simulink model "lump_model_v9"  (R2024b)
settings: Solver=FixedStepAuto  StartTime=0.0  StopTime=100  FixedStep=0.001  RelTol=1e-3
model workspace (MAT data in the model file):
  A_busbar = 0.0015
  A_pack = 0.711626248
  C_nominal = 3
  I_max = 157.708978328
  P = 5
  S = 138
  SoC_initial = 0.78
  T_amb = 297.15
  W_max = 34
  busbar_CC_area = 0.000108
  busbar_Cp = 237
  busbar_length = 0.032
  busbar_mass = 0.01
  busbar_resistivity = 1.68e-08
  busbar_thermalcontact_resistance = 1
  cell_Cp = 1000
  cell_mass = 0.046
  h_busbar = 5
  h_pack = 5
libraries: nesl_utility x8, fl_lib x6, ee_lib x2
settings Model: Creator=kara.28  LastModifiedBy=account

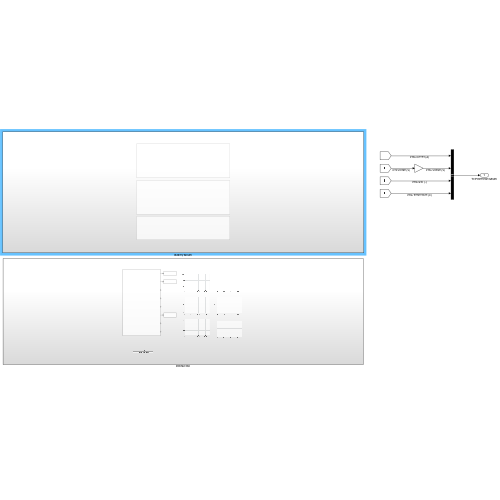
[thumbnail: Simulink's stored preview of the top-level diagram]
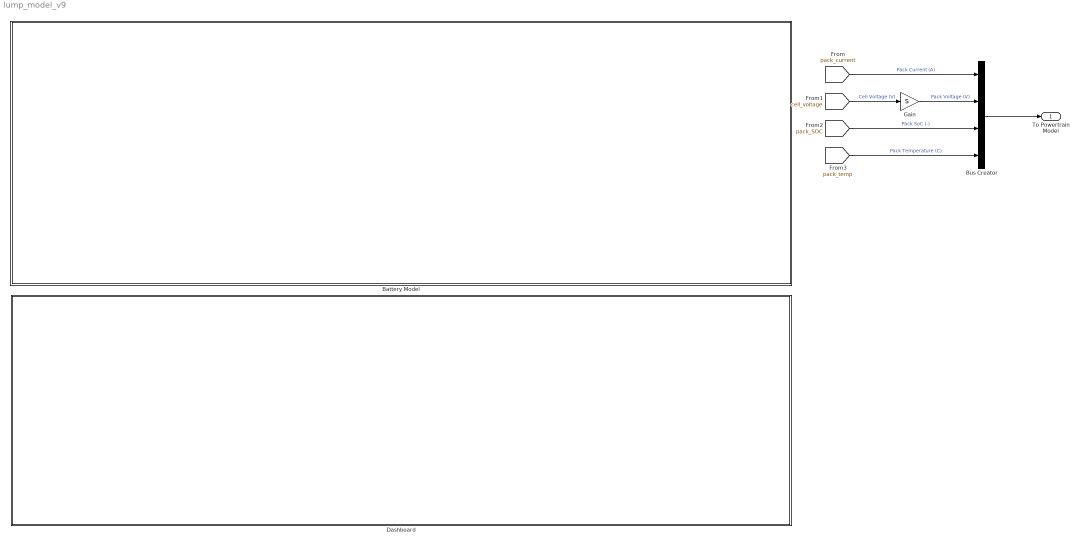
== system lump_model_v9 ==
  Battery Model : Subsystem
  Bus Creator : BusCreator  Inputs=4
  Dashboard : Subsystem
  Gain : Gain  Gain=S
  To Powertrain Model : Outport
  wires:
  [pack_temp] -> Bus Creator/4  "Pack Temperature (C)"
  [pack_SOC] -> Bus Creator/3  "Pack SoC (-)"
  [cell_voltage] -> Gain/1  "Cell Voltage (V)"
  [pack_current] -> Bus Creator/1  "Pack Current (A)"
  Gain/1 -> Bus Creator/2  "Pack Voltage (V)"
  Bus Creator/1 -> To Powertrain Model/1

== system lump_model_v9/Battery Model ==
  Air Temp : Subsystem
  Battery Cells : Subsystem
  Bus Bars : Subsystem

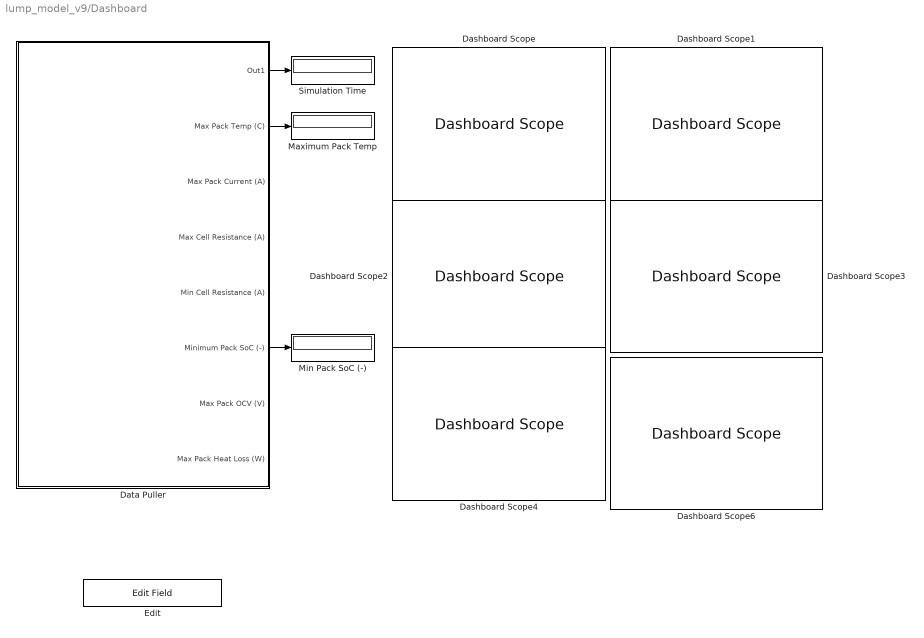
== system lump_model_v9/Dashboard ==
  Dashboard Scope : DashboardScope  Ymin=35  Ymax=60
  Dashboard Scope1 : DashboardScope  Ymin=0  Ymax=180
  Dashboard Scope2 : DashboardScope
  Dashboard Scope3 : DashboardScope  Ymin=0  Ymax=1
  Dashboard Scope4 : DashboardScope  Ymin=2.5  Ymax=4.2
  Dashboard Scope6 : DashboardScope
  Data Puller : Subsystem
  Edit : EditField  ShowInitialText=on  Alignment=Center
  Maximum Pack Temp : Display
  Min Pack SoC (-) : Display
  Simulation Time : Display
  wires:
  Data Puller/1(Out1) -> Simulation Time/1
  Data Puller/2(Max Pack Temp (C)) -> Maximum Pack Temp/1
  Data Puller/6(Minimum Pack SoC (-)) -> Min Pack SoC (-)/1

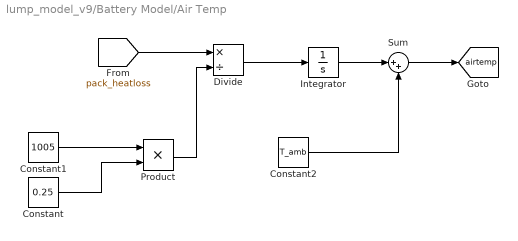
== system lump_model_v9/Battery Model/Air Temp ==
  Constant : Constant  Value=0.25
  Constant1 : Constant  Value=1005
  Constant2 : Constant  Value=T_amb
  Divide : Product  Inputs=*/
  Integrator : Integrator
  Product : Product
  Sum : Sum  Inputs=|++
  tag scope: airtemp=global
  wires:
  [pack_heatloss] -> Divide/1
  Product/1 -> Divide/2
  Constant/1 -> Product/2
  Constant1/1 -> Product/1
  Divide/1 -> Integrator/1
  Integrator/1 -> Sum/1
  Constant2/1 -> Sum/2
  Sum/1 -> [airtemp]

== system lump_model_v9/Battery Model/Battery Cells ==
  Battery Heat : Subsystem
      settings: PortSchema="{\"entries\":[{\"content\":{\"sides\":[{\"content\":{\"connectorIds\":[\"In1\",\"Out1\",\"In2\"]},\"type\":\"ConnectorPlacement.EquallySpacedRectSide\",\"uuid\":\"0f7c0562-63f7-413a-9c65-7d5d0f23ac53\"},{\"content\":{\"side\":\"RIGHT\"},\"type\":\"ConnectorPlacement.EquallySpacedRectSide\",\"uuid\":\"6856fc4a-e601-47fb-aafe-3183d6398fa2\"},{\"content\":{\"side\":\"TOP\"},\"type\":\"ConnectorPlacement.EquallySpacedRectSide\",\"uuid\":\"93500152-ab0c-4e86-a765-8796b82b9cd6\"}]},\"type\":\"ConnectorPlacement.EquallySpacedConnector\",\"uuid\":\"8bef09a8-0835-4033-ba4e-3f5f6277d0ac\"}],\"packageUris\":[\"http://schema.mathworks.com/mf0/Connector/R2020b\"],\"version\":\"1.0\"}"
  Battery Heat Generation : Subsystem
  Heat Loss : Subsystem
      settings: PortSchema="{\"entries\":[{\"content\":{\"sides\":[{\"content\":{},\"type\":\"ConnectorPlacement.EquallySpacedRectSide\",\"uuid\":\"cd11f8f0-ebc0-4dda-8c98-00f5919de41a\"},{\"content\":{\"connectorIds\":[\"In1\",\"Out1\"],\"side\":\"RIGHT\"},\"type\":\"ConnectorPlacement.EquallySpacedRectSide\",\"uuid\":\"2a68a9a1-bd97-4a17-8a8b-1aa98e9bd9a8\"},{\"content\":{\"side\":\"TOP\"},\"type\":\"ConnectorPlacement.EquallySpacedRectSide\",\"uuid\":\"debcc510-941b-4448-a371-f67c84c59f32\"}]},\"type\":\"ConnectorPlacement.EquallySpacedConnector\",\"uuid\":\"91559e46-754b-48b4-ac3e-ab135f9add0a\"}],\"packageUris\":[\"http://schema.mathworks.com/mf0/Connector/R2020b\"],\"version\":\"1.0\"}"
  wires:
  Battery Heat/1(Pack Temp (K)) -> Heat Loss/1(Pack Temp (K))
  Battery Heat Generation/1(Battery Heat Generation Rate) -> Battery Heat/1(Battery Heat Generation)
  Heat Loss/1(Pack Heat Loss Rate) -> Battery Heat/2(Battery Heat Loss)

== system lump_model_v9/Battery Model/Bus Bars ==
  Ambient Heat Loss : Subsystem
      settings: PortSchema="{\"entries\":[{\"content\":{\"sides\":[{\"content\":{},\"type\":\"ConnectorPlacement.EquallySpacedRectSide\",\"uuid\":\"cd11f8f0-ebc0-4dda-8c98-00f5919de41a\"},{\"content\":{\"connectorIds\":[\"In1\",\"Out1\"],\"side\":\"RIGHT\"},\"type\":\"ConnectorPlacement.EquallySpacedRectSide\",\"uuid\":\"2a68a9a1-bd97-4a17-8a8b-1aa98e9bd9a8\"},{\"content\":{\"side\":\"TOP\"},\"type\":\"ConnectorPlacement.EquallySpacedRectSide\",\"uuid\":\"debcc510-941b-4448-a371-f67c84c59f32\"}]},\"type\":\"ConnectorPlacement.EquallySpacedConnector\",\"uuid\":\"91559e46-754b-48b4-ac3e-ab135f9add0a\"}],\"packageUris\":[\"http://schema.mathworks.com/mf0/Connector/R2020b\"],\"version\":\"1.0\"}"
  Busbar Heat : Subsystem
      settings: PortSchema="{\"entries\":[{\"content\":{\"sides\":[{\"content\":{\"connectorIds\":[\"In1\",\"Out1\",\"In2\"]},\"type\":\"ConnectorPlacement.EquallySpacedRectSide\",\"uuid\":\"0f7c0562-63f7-413a-9c65-7d5d0f23ac53\"},{\"content\":{\"side\":\"RIGHT\"},\"type\":\"ConnectorPlacement.EquallySpacedRectSide\",\"uuid\":\"6856fc4a-e601-47fb-aafe-3183d6398fa2\"},{\"content\":{\"side\":\"TOP\"},\"type\":\"ConnectorPlacement.EquallySpacedRectSide\",\"uuid\":\"93500152-ab0c-4e86-a765-8796b82b9cd6\"}]},\"type\":\"ConnectorPlacement.EquallySpacedConnector\",\"uuid\":\"8bef09a8-0835-4033-ba4e-3f5f6277d0ac\"}],\"packageUris\":[\"http://schema.mathworks.com/mf0/Connector/R2020b\"],\"version\":\"1.0\"}"
  Resistance Heat Generation : Subsystem
  wires:
  Ambient Heat Loss/1(Busbar Heat Loss Rate) -> Busbar Heat/2(Busbar Heat Loss)
  Resistance Heat Generation/1(Busbar Heat Generation Rate) -> Busbar Heat/1(Busbar Heat Generation)
  Busbar Heat/1(Busbar Temp (K)) -> Ambient Heat Loss/1(Busbar Temp (K))

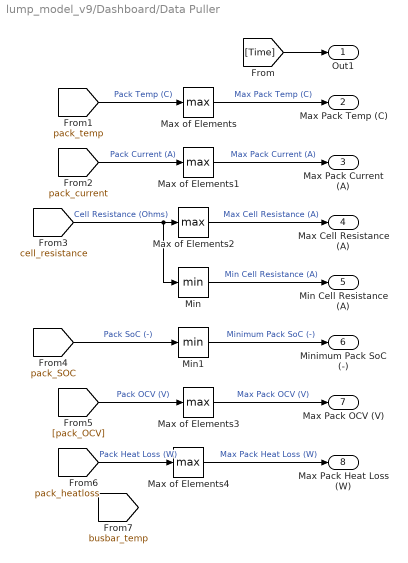
== system lump_model_v9/Dashboard/Data Puller ==
  Max of Elements{,1..4} (5 alike) : MinMax  Function=max
  Min : MinMax
  Min1 : MinMax
  Out1 : Outport
  Max Pack Temp (C) : Outport  Port=2
  Max Pack Current (A) : Outport  Port=3
  Max Cell Resistance (A) : Outport  Port=4
  Min Cell Resistance (A) : Outport  Port=5
  Minimum Pack SoC (-) : Outport  Port=6
  Max Pack OCV (V) : Outport  Port=7
  Max Pack Heat Loss (W) : Outport  Port=8
  wires:
  Min1/1 -> Minimum Pack SoC (-)/1  "Minimum Pack SoC (-)"
  [pack_current] -> Max of Elements1/1  "Pack Current (A)"
  [cell_resistance] -> Min/1, Max of Elements2/1  "Cell Resistance (Ohms)"
  [pack_heatloss] -> Max of Elements4/1  "Pack Heat Loss (W)"
  [pack_temp] -> Max of Elements/1  "Pack Temp (C)"
  [pack_OCV] -> Max of Elements3/1  "Pack OCV (V)"
  [pack_SOC] -> Min1/1  "Pack SoC (-)"
  Max of Elements1/1 -> Max Pack Current (A)/1  "Max Pack Current (A)"
  Max of Elements2/1 -> Max Cell Resistance (A)/1  "Max Cell Resistance (A)"
  Max of Elements/1 -> Max Pack Temp (C)/1  "Max Pack Temp (C)"
  Max of Elements4/1 -> Max Pack Heat Loss (W)/1  "Max Pack Heat Loss (W)"
  Max of Elements3/1 -> Max Pack OCV (V)/1  "Max Pack OCV (V)"
  [Time] -> Out1/1
  Min/1 -> Min Cell Resistance (A)/1  "Min Cell Resistance (A)"

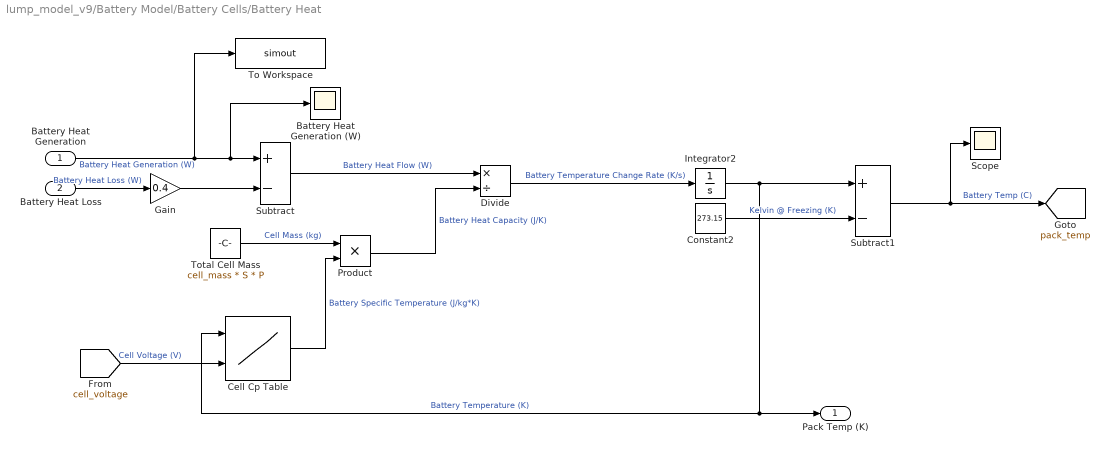
== system lump_model_v9/Battery Model/Battery Cells/Battery Heat ==
  Battery Heat Generation : Inport
  Battery Heat Loss : Inport  Port=2
  Battery Heat Generation (W) : Scope
  Cell Cp Table : Lookup_n-D  BreakpointsForDimension1=[296.0488;303.3425;312.147;321.5769;330.6423]  BreakpointsForDimension2=[0 0.5 1]  Table=[811.0868 819.6535 830.8545;814.1373 822.704 834.6964;817.9826 826.8129 838.6737000000001;822.2249 831.0552 843.4446;826.7299 835.8239 848.3459]  InterpMethod=Cubic spline  InternalRulePriority=Speed  RndMeth=Simplest
      settings: InputPortMap=u0,u1
  Constant2 : Constant  Value=273.15
  Divide : Product  Inputs=*/
  Gain : Gain  Gain=0.4
  Integrator2 : Integrator  InitialCondition=T_amb
  Product : Product
  Scope : Scope
  Subtract : Sum  Inputs=+-
  Subtract1 : Sum  Inputs=+-
  To Workspace : ToWorkspace  VariableName=simout  SampleTime=-1
  Total Cell Mass : Constant  Value=cell_mass * S * P
  Pack Temp (K) : Outport
  tag scope: pack_temp=global
  wires:
  Cell Cp Table/1 -> Product/2  "Battery Specific Temperature (J/kg*K)"
  Constant2/1 -> Subtract1/2  "Kelvin @ Freezing (K)"
  Divide/1 -> Integrator2/1  "Battery Temperature Change Rate (K/s)"
  Subtract/1 -> Divide/1  "Battery Heat Flow (W)"
  Integrator2/1 -> Cell Cp Table/1, Pack Temp (K)/1, Subtract1/1  "Battery Temperature (K)"
  Subtract1/1 -> Scope/1, [pack_temp]  "Battery Temp (C)"
  Total Cell Mass/1 -> Product/1  "Cell Mass (kg)"
  Product/1 -> Divide/2  "Battery Heat Capacity (J/K)"
  Battery Heat Loss/1 -> Gain/1  "Battery Heat Loss (W)"
  Battery Heat Generation/1 -> To Workspace/1, Battery Heat Generation (W)/1, Subtract/1  "Battery Heat Generation (W)"
  [cell_voltage] -> Cell Cp Table/2  "Cell Voltage (V)"
  Gain/1 -> Subtract/2

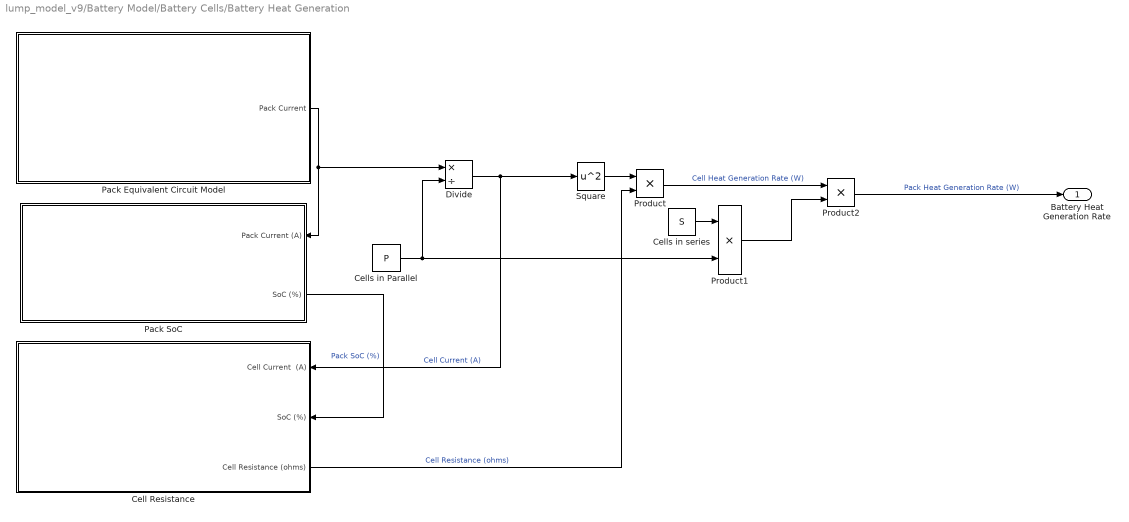
== system lump_model_v9/Battery Model/Battery Cells/Battery Heat Generation ==
  Cell Resistance : Subsystem
      settings: PortSchema="{\"entries\":[{\"content\":{\"sides\":[{\"content\":{},\"type\":\"ConnectorPlacement.EquallySpacedRectSide\",\"uuid\":\"1c6ff2a8-2c86-4b92-aa7d-5717a02d6f28\"},{\"content\":{\"connectorIds\":[\"In1\",\"In2\",\"Out1\"],\"side\":\"RIGHT\"},\"type\":\"ConnectorPlacement.EquallySpacedRectSide\",\"uuid\":\"52a4cb2c-e1db-459d-bd0a-206cc3bba6d1\"},{\"content\":{\"side\":\"TOP\"},\"type\":\"ConnectorPlacement.EquallySpacedRectSide\",\"uuid\":\"751bbbd6-abc7-4265-8d68-4aa70d69379f\"}]},\"type\":\"ConnectorPlacement.EquallySpacedConnector\",\"uuid\":\"b8f9630f-0167-4478-8d98-637e13782dcd\"}],\"packageUris\":[\"http://schema.mathworks.com/mf0/Connector/R2020b\"],\"version\":\"1.0\"}"
      mask Display: image('resistor.png');
  Cells in Parallel : Constant  Value=P
  Cells in series : Constant  Value=S
  Divide : Product  Inputs=*/
  Pack Equivalent Circuit Model : Subsystem
      mask Display: image('current.png');
  Pack SoC : Subsystem
      settings: PortSchema="{\"entries\":[{\"content\":{\"sides\":[{\"content\":{},\"type\":\"ConnectorPlacement.EquallySpacedRectSide\",\"uuid\":\"1c6ff2a8-2c86-4b92-aa7d-5717a02d6f28\"},{\"content\":{\"connectorIds\":[\"In1\",\"Out1\"],\"side\":\"RIGHT\"},\"type\":\"ConnectorPlacement.EquallySpacedRectSide\",\"uuid\":\"52a4cb2c-e1db-459d-bd0a-206cc3bba6d1\"},{\"content\":{\"side\":\"TOP\"},\"type\":\"ConnectorPlacement.EquallySpacedRectSide\",\"uuid\":\"751bbbd6-abc7-4265-8d68-4aa70d69379f\"}]},\"type\":\"ConnectorPlacement.EquallySpacedConnector\",\"uuid\":\"b8f9630f-0167-4478-8d98-637e13782dcd\"}],\"packageUris\":[\"http://schema.mathworks.com/mf0/Connector/R2020b\"],\"version\":\"1.0\"}"
      mask Display: image('SoC.jpg');
  Product : Product
  Product1 : Product
  Product2 : Product
  Square : Math  Operator=square
  Battery Heat Generation Rate : Outport
  wires:
  Cells in series/1 -> Product1/1
  Divide/1 -> Cell Resistance/1(Cell Current  (A)), Square/1  "Cell Current (A)"
  Cell Resistance/1(Cell Resistance (ohms)) -> Product/2  "Cell Resistance (ohms)"
  Square/1 -> Product/1
  Cells in Parallel/1 -> Divide/2, Product1/2
  Product1/1 -> Product2/2
  Product/1 -> Product2/1  "Cell Heat Generation Rate (W)"
  Product2/1 -> Battery Heat Generation Rate/1  "Pack Heat Generation Rate (W)"
  Pack SoC/1(SoC (%)) -> Cell Resistance/2(SoC (%))  "Pack SoC (%)"
  Pack Equivalent Circuit Model/1(Pack Current) -> Divide/1, Pack SoC/1(Pack Current (A))

== system lump_model_v9/Battery Model/Battery Cells/Heat Loss ==
  Pack Temp (K) : Inport
  Pack Convective Heat Transfer Coefficient (W/m^2*K) : Constant  Value=h_pack
  Pack Surface Area (m^2) : Gain  Gain=A_pack
  Product : Product
  Subtract : Sum  Inputs=+-
  Pack Heat Loss Rate : Outport
  tag scope: pack_heatloss=global
  wires:
  Pack Convective Heat Transfer Coefficient (W/m^2*K)/1 -> Pack Surface Area (m^2)/1  "Pack Convective Heat Transfer Coefficient (W/m^2*K)"
  Subtract/1 -> Product/2  "Temperature Difference (K)"
  Pack Surface Area (m^2)/1 -> Product/1  "Heat Transfer Capacitance (W/K)"
  Product/1 -> [pack_heatloss], Pack Heat Loss Rate/1  "Pack Heat Loss Rate (W)"
  Pack Temp (K)/1 -> Subtract/1  "Pack Temp (K)"
  [airtemp] -> Subtract/2  "Ambient Temp (K)"

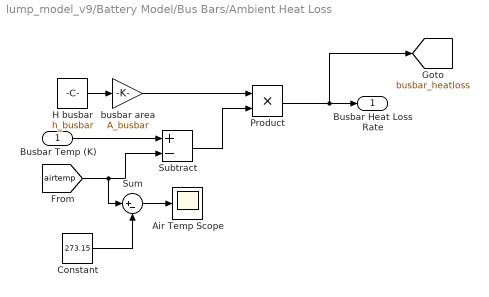
== system lump_model_v9/Battery Model/Bus Bars/Ambient Heat Loss ==
  Busbar Temp (K) : Inport
  Air Temp Scope : Scope
  Constant : Constant  Value=273.15
  H busbar : Constant  Value=h_busbar
  Product : Product
  Subtract : Sum  Inputs=+-
  Sum : Sum  Inputs=|+-
  busbar area : Gain  Gain=A_busbar
  Busbar Heat Loss Rate : Outport
  tag scope: busbar_heatloss=global
  wires:
  [airtemp] -> Sum/1, Subtract/2
  Busbar Temp (K)/1 -> Subtract/1
  Product/1 -> Busbar Heat Loss Rate/1, [busbar_heatloss]
  busbar area/1 -> Product/1
  Subtract/1 -> Product/2
  H busbar/1 -> busbar area/1
  Sum/1 -> Air Temp Scope/1
  Constant/1 -> Sum/2

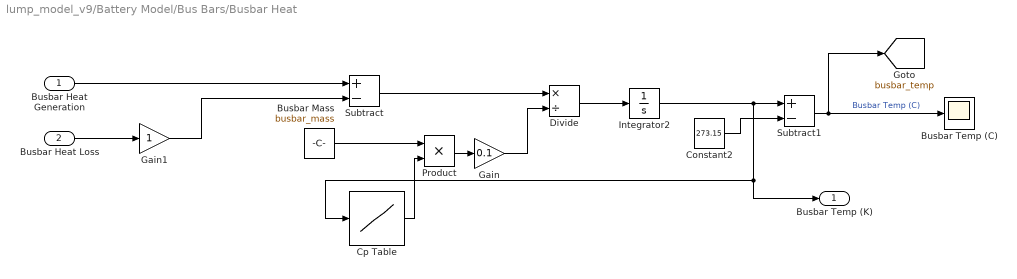
== system lump_model_v9/Battery Model/Bus Bars/Busbar Heat ==
  Busbar Heat Generation : Inport
  Busbar Heat Loss : Inport  Port=2
  Busbar Mass : Constant  Value=busbar_mass
  Busbar Temp (C) : Scope
  Constant2 : Constant  Value=273.15
  Cp Table : Lookup_n-D  NumberOfTableDimensions=1  BreakpointsForDimension1=[300;400;600;800;1000]  Table=[401;393;379;366;352]  InterpMethod=Cubic spline  InternalRulePriority=Speed  RndMeth=Simplest
  Divide : Product  Inputs=*/
  Gain : Gain  Gain=0.1
  Gain1 : Gain
  Integrator2 : Integrator  InitialCondition=T_amb
  Product : Product
  Subtract : Sum  Inputs=+-
  Subtract1 : Sum  Inputs=+-
  Busbar Temp (K) : Outport
  tag scope: busbar_temp=global
  wires:
  Product/1 -> Gain/1
  Busbar Mass/1 -> Product/1
  Subtract1/1 -> Busbar Temp (C)/1, [busbar_temp]  "Busbar Temp (C)"
  Integrator2/1 -> Subtract1/1, Busbar Temp (K)/1, Cp Table/1
  Subtract/1 -> Divide/1
  Divide/1 -> Integrator2/1
  Constant2/1 -> Subtract1/2
  Cp Table/1 -> Product/2
  Busbar Heat Generation/1 -> Subtract/1
  Gain/1 -> Divide/2
  Busbar Heat Loss/1 -> Gain1/1
  Gain1/1 -> Subtract/2

== system lump_model_v9/Battery Model/Bus Bars/Resistance Heat Generation ==
  Busbar cross sectional area (m^2) : Constant  Value=busbar_CC_area
  Busbar length (m) : Constant  Value=busbar_length
  Busbar resistivity (Ohms * m) : Constant  Value=busbar_resistivity
  Divide : Product  Inputs=*/
  Product : Product
  Product1 : Product
  Square : Math  Operator=square
  Busbar Heat Generation Rate : Outport
  wires:
  Divide/1 -> Product/2  "Busbar resistance (ohms)"
  Busbar cross sectional area (m^2)/1 -> Divide/2
  Product1/1 -> Divide/1
  Busbar length (m)/1 -> Product1/2
  Busbar resistivity (Ohms * m)/1 -> Product1/1
  Square/1 -> Product/1
  [pack_current] -> Square/1  "Pack Current (A)"
  Product/1 -> Busbar Heat Generation Rate/1  "Busbar Heat Gain (W)"

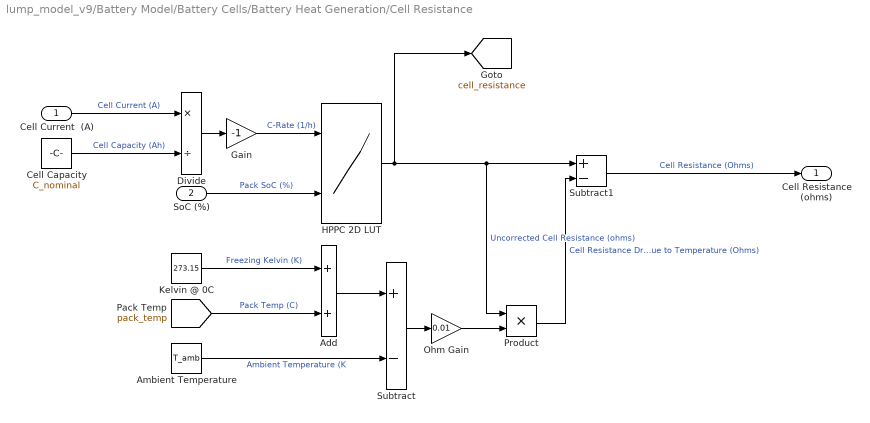
== system lump_model_v9/Battery Model/Battery Cells/Battery Heat Generation/Cell Resistance ==
  Cell Current  (A) : Inport
  SoC (%) : Inport  Port=2
  Add : Sum
  Ambient Temperature : Constant  Value=T_amb
  Cell Capacity : Constant  Value=C_nominal
  Divide : Product  Inputs=*/
  Gain : Gain  Gain=-1
  HPPC 2D LUT : Lookup_n-D  BreakpointsForDimension1=[-10;-5;-1;1;2;3]  BreakpointsForDimension2=[0.1;0.2;0.3;0.4;0.5;0.6;0.7;0.8;0.9;1]  Table=[0.018906 0.01868 0.018453 0.018226 0.017999 0.017916 0.017743 0.018183 0.019549 0.022703;0.021356 0.020344 0.019332 0.019017 0.018694 0.018598 0.018319 0.018773 0.020642 0.024917;0.02305 0.020909 0.018859 0.019644 0.019687 0.018989 0.018291 0.019295 0.021608 0.026536;0.023001 0.020599 0.019683 0.019161 0.01894 0.018506 0.018636 0.019336 0.020993 0.02265;0.022654 0.020712 0.018901 0.018682 0.018442 0.018289 0.017788 0.017286 0.016785 0.016283;0.019898 0.017891 0.017366 0.01725 0.01725 0.017251 0.017251 0.017251 0.017251 0.017251]  InterpMethod=Cubic spline  ExtrapMethod=Clip  InternalRulePriority=Speed  RndMeth=Simplest
      settings: InputPortMap=u0,u1
  Kelvin @ 0C : Constant  Value=273.15
  Ohm Gain : Gain  Gain=0.01
  Product : Product
  Subtract : Sum  Inputs=+-
  Subtract1 : Sum  Inputs=+-
  Cell Resistance (ohms) : Outport
  tag scope: cell_resistance=global
  wires:
  Cell Current  (A)/1 -> Divide/1  "Cell Current (A)"
  Cell Capacity/1 -> Divide/2  "Cell Capacity (Ah)"
  SoC (%)/1 -> HPPC 2D LUT/2  "Pack SoC (%)"
  HPPC 2D LUT/1 -> [cell_resistance], Subtract1/1, Product/1  "Uncorrected Cell Resistance (ohms)"
  Divide/1 -> Gain/1
  Gain/1 -> HPPC 2D LUT/1  "C-Rate (1/h)"
  Subtract/1 -> Ohm Gain/1
  Ambient Temperature/1 -> Subtract/2  "Ambient Temperature (K"
  [pack_temp] -> Add/2  "Pack Temp (C)"
  Add/1 -> Subtract/1
  Kelvin @ 0C/1 -> Add/1  "Freezing Kelvin (K)"
  Ohm Gain/1 -> Product/2
  Product/1 -> Subtract1/2  "Cell Resistance Drop Due to Temperature (Ohms)"
  Subtract1/1 -> Cell Resistance (ohms)/1  "Cell Resistance (Ohms)"

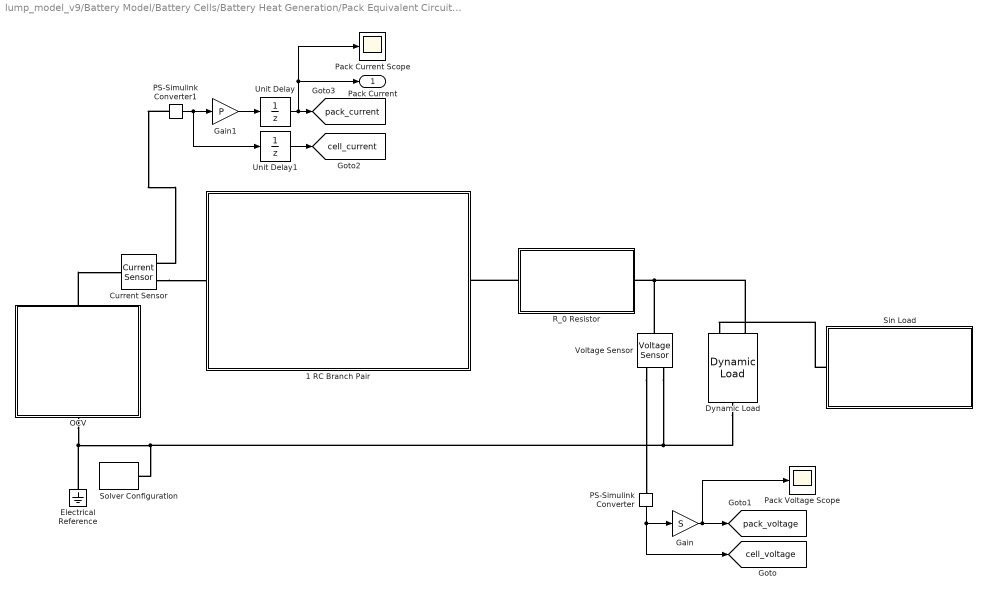
== system lump_model_v9/Battery Model/Battery Cells/Battery Heat Generation/Pack Equivalent Circuit Model ==
  1 RC Branch Pair : Subsystem
  Current Sensor : fl_lib/Electrical/Electrical Sensors/Current Sensor
  Dynamic Load : ee_lib/Passive/Dynamic Load  load_type=ee.enum.dc_ac.dc  min_supply_voltage=20 V  pow_min=1e-3 W  G_reverse=1e-6 S  deltaV=1e-3 V  f0=60 Hz  Vrms_min=200 V  tau=0.01 s  Vrms_ini=300 V  Vang_ini=0 deg  fault_action=simscape.enum.assert.action.none  t_fault=1 s
      settings: InternalSimscapePortConfiguration="{\"Bottom\":[],\"Left\":[{\"id\":\"p\",\"label\":\"+\",\"type\":\"foundation.electrical.electrical\"}],\"Right\":[{\"id\":\"n\",\"label\":\"-\",\"type\":\"foundation.electrical.electrical\"}],\"Top\":[{\"id\":\"P\",\"label\":\"P\",\"type\":\"input\"}]}"
  Electrical Reference : fl_lib/Electrical/Electrical Elements/Electrical Reference
  Gain : Gain  Gain=S
  Gain1 : Gain  Gain=P
  OCV : Subsystem
  PS-Simulink Converter : nesl_utility/PS-Simulink Converter  PhysicalDomain=network_engine_domain  SubClassName=ps_output  LeftPortType=input  RightPortType=output  PseudoPeriodic=off  Frequencies=[]  VectorFormat=inherit  Unit=inherit  AffineConversion=off
  PS-Simulink Converter1 : nesl_utility/PS-Simulink Converter  PhysicalDomain=network_engine_domain  SubClassName=ps_output  LeftPortType=input  RightPortType=output  PseudoPeriodic=off  Frequencies=[]  VectorFormat=inherit  Unit=inherit  AffineConversion=off
  Pack Current Scope : Scope
  Pack Voltage Scope : Scope
  R_0 Resistor : Subsystem
  Sin Load : Subsystem
  Solver Configuration : nesl_utility/Solver Configuration  PhysicalDomain=network_engine_domain  SubClassName=solver  LeftPortType=input  RightPortType=generic  Tones=[]  Harmonics=[]  SimulateNoise=off  Profile=off  UseLocalSampling=off  EnableSwitchedLinearOptims=on  FrequencyDomain=off  UseCCode=off  RelTol=0.001  AbsTol=0.001  MinStep=1e-09  ToWorkspace=off  RevertToSquareIcSolve=off  NumHomotopyIterations=100  PhasorMode=off  PhasorModeNumHarmonics=1  ConsistencySolver=NEWTON_XTOL_AFTER_FTOL  IndexReductionMethod=DerivativeReplacement  DoDC=off  ResidualTolerance=1e-09  ConsistencyTolSource=GLOBAL  ConsistencyAbsTol=0.001  ConsistencyRelTol=0.001  ConsistencyTolFactor=0.001  UseLocalSolver=off  LocalSolverChoice=NE_BACKWARD_EULER_ADVANCER  ResolveIndetEquations=on  FunctionEvalNumThread=1  LocalSolverSampleTime=0.001  DoFixedCost=off  MaxNonlinIter=3  MaxModeIter=2  ComputeImpulses=off  ImpulseIterations=2  LinearAlgebra=auto  LinearAlgebraNumThread=0  EquationFormulation=NE_TIME_EF  DelaysMemoryBudget=1024  AutomaticFiltering=on  FilteringTimeConstant=0.001  PartitionStorageMethod=AS_NEEDED  PartitionMemoryBudget=1024  PartitionMethod=ROBUST  MultibodyUseLocalSolver=off  MultibodyLocalSolverChoice=ODE1  MultibodyLocalSolverSampleTime=0.001
  Unit Delay : UnitDelay  SampleTime=-1  HasFrameUpgradeWarning=on
  Unit Delay1 : UnitDelay  SampleTime=-1  HasFrameUpgradeWarning=on
  Voltage Sensor : fl_lib/Electrical/Electrical Sensors/Voltage Sensor
  Pack Current : Outport
  tag scope: cell_current=global, cell_voltage=global, pack_current=global, pack_voltage=global
  wires:
  Gain/1 -> [pack_voltage], Pack Voltage Scope/1
  Gain1/1 -> Unit Delay/1
  Unit Delay1/1 -> [cell_current]
  Unit Delay/1 -> Pack Current Scope/1, Pack Current/1, [pack_current]
  PS-Simulink Converter1/1 -> Unit Delay1/1, Gain1/1
  PS-Simulink Converter/1 -> Gain/1, [cell_voltage]
  connections:
  R_0 Resistor/LConn1 -- 1 RC Branch Pair/RConn1
  Voltage Sensor/RConn1 -- PS-Simulink Converter/LConn1
  OCV/RConn1 -- Dynamic Load/RConn1 -- Voltage Sensor/RConn2 -- Solver Configuration/RConn1 -- Electrical Reference/LConn1
  PS-Simulink Converter1/LConn1 -- Current Sensor/RConn1
  Voltage Sensor/LConn1 -- R_0 Resistor/RConn1 -- Dynamic Load/LConn1
  Sin Load/RConn1 -- Dynamic Load/LConn2
  OCV/LConn1 -- Current Sensor/LConn1
  Current Sensor/RConn2 -- 1 RC Branch Pair/LConn1

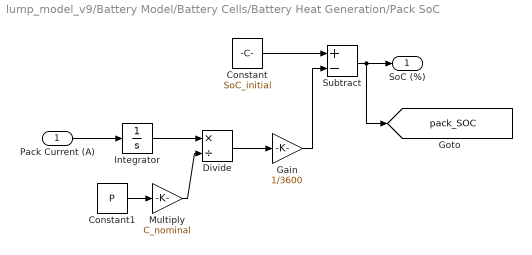
== system lump_model_v9/Battery Model/Battery Cells/Battery Heat Generation/Pack SoC ==
  Pack Current (A) : Inport
  Constant : Constant  Value=SoC_initial
  Constant1 : Constant  Value=P
  Divide : Product  Inputs=*/
  Gain : Gain  Gain=1/3600
  Integrator : Integrator
  Multiply : Gain  Gain=C_nominal
  Subtract : Sum  Inputs=+-
  SoC (%) : Outport
  tag scope: pack_SOC=global
  wires:
  Pack Current (A)/1 -> Integrator/1
  Constant/1 -> Subtract/1
  Integrator/1 -> Divide/1
  Subtract/1 -> [pack_SOC], SoC (%)/1
  Constant1/1 -> Multiply/1
  Multiply/1 -> Divide/2
  Divide/1 -> Gain/1
  Gain/1 -> Subtract/2

== system lump_model_v9/Battery Model/Battery Cells/Battery Heat Generation/Pack Equivalent Circuit Model/1 RC Branch Pair ==
  Capacitor : Subsystem
  Resistor : Subsystem
  RC Output : PMIOPort  Side=Right
  RC Input : PMIOPort  Port=2  Side=Left
  connections:
  Capacitor/LConn1 -- Resistor/LConn1 -- RC Input/RConn1
  Resistor/RConn1 -- Capacitor/RConn1 -- RC Output/RConn1

== system lump_model_v9/Battery Model/Battery Cells/Battery Heat Generation/Pack Equivalent Circuit Model/OCV ==
  2-D Lookup Table : Lookup_n-D  BreakpointsForDimension1=[25 40 60]  BreakpointsForDimension2=[0;0.10000000000000001;0.20000000000000001;0.29999999999999999;0.40000000000000002;0.5;0.59999999999999998;0.69999999999999996;0.80000000000000004;0.90000000000000002]  Table=[4.1899733543396 4.09245538711548 4.04466485977173 3.93737483024597 3.83577251434326 3.75628757476807 3.66292858123779 3.53464698791504 3.44169187545776 3.23304915428162;4.19153022766113 4.09326219558716 4.04607534408569 3.93875551223755 3.83869075775147 3.75923085212708 3.65240955352783 3.5323486328125 3.44081568717957 3.22783327102661;4.1908655166626 4.09230852127075 4.04864549636841 3.9411768913269 3.84473943710327 3.7643346786499 3.64451742172241 3.529953956604 3.43093800544739 3.2243959903717]  InterpMethod=Cubic spline  InternalRulePriority=Speed  RndMeth=Simplest
      settings: InputPortMap=u0,u1
  OCV : fl_lib/Electrical/Electrical Sources/Controlled Voltage Source
  Simulink-PS Converter : nesl_utility/Simulink-PS Converter  PhysicalDomain=network_engine_domain  SubClassName=ps_input  LeftPortType=input  RightPortType=output  PseudoPeriodic=off  Frequencies=[]  NoiseDistribution=none  NoiseParameters=[]  Unit=V  AffineConversion=off  FilteringAndDerivatives=provide  SimscapeFilterOrder=1  InputFilterTimeConstant=0.001  UdotUserProvided=0
  SoC deployed calculator : Subsystem
  OCV Output : PMIOPort  Side=Left
  OCV Input : PMIOPort  Port=2  Side=Right
  wires:
  [pack_temp] -> 2-D Lookup Table/1  "Battery Temp (C)"
  2-D Lookup Table/1 -> Simulink-PS Converter/1
  SoC deployed calculator/1(SoC Used (-)) -> 2-D Lookup Table/2  "SoC Used (-)"
  connections:
  OCV/RConn2 -- OCV Input/RConn1
  OCV/LConn1 -- OCV Output/RConn1
  Simulink-PS Converter/RConn1 -- OCV/RConn1

== system lump_model_v9/Battery Model/Battery Cells/Battery Heat Generation/Pack Equivalent Circuit Model/R_0 Resistor ==
  3-D Lookup Table : Lookup_n-D  NumberOfTableDimensions=3  BreakpointsForDimension1=[0 0.10000000000000001 0.20000000000000001 0.29999999999999999 0.40000000000000002 0.5 0.59999999999999998 0.69999999999999996 0.80000000000000004 0.90000000000000002]  BreakpointsForDimension2=[25 40 60]  BreakpointsForDimension3=[-9.61780450282953 -4.80898979382637 -0.960911970872145 -0.320367568578476 0.322065353393555 0.963286375388121 1.60506175114558 1.92546795576047]  Table=reshape([0.0208969457515545 0.0185429568837496 0.0175689631975861 0.0171342767590725 0.0170817865790692 0.0170273088031529 0.0171672542375037 0.0171672542375037 0.0171672542375037 0.0171672542375037 0.016375134849274 0.0148030322913059 0.014244238055347 0.0139370990131393 0.0138742447759964 0.0138774461382894 0.0139075954925356 0.0140718169046758 0.0140718169046758 0.0140718169046758 0.0143655689080314 0.0133457294428562 0.0129696195510676 0.0127699129139726 0.0127151882120239 0.012722766072234 0.0127425113124588 0.0128371552499186 0.0130748389191311 0.0130748389191311 0.0223977468803507 0.0192561093239405 0.0181700779776692 0.017576759274244 0.0173983350854821 0.0174117696520015 0.017495915689451 0.017741061324451 0.0186485051759371 0.0186485051759371 0.016838892362239 0.0150452279742284 0.0144124859184527 0.0140465382415619 0.0139281588595513 0.0139027427376644 0.0139328084610531 0.0140816570296377 0.0145628596541215 0.0157854264637026 0.0145216387506235 0.0134470763585342 0.0130677705542268 0.0128148983747903 0.0126999024124993 0.0127036172567835 0.0127328717553446 0.0128107916443252 0.0131412786384986 0.013868894910505 0.0235781019610261 0.0196857777097367 0.0184860233386763 0.0177959603366917 0.0175525262870582 0.0175685448471578 0.017591973414872 0.0178880498713393 0.0187796463236645 0.0209952384417786 0.0173346905030945 0.0151268573513354 0.0144851969150989 0.0141172832970184 0.0139044596304346 0.0139036185838405 0.0139185877290097 0.0140954894433781 0.0145442950262368 0.015744162170302 0.0148705562433675 0.0134984179313018 0.0131082225464489 0.0128894594904751 0.0127070850388396 0.0127061718881569 0.0127130968113931 0.0128154860955142 0.0131027489213916 0.013888427958746 0.0246442754506806 0.0197474595379293 0.0183374118574875 0.0177337520090252 0.0175833108212411 0.0175271613187289 0.0174864168184484 0.0179466248858059 0.0187984050043328 0.0209514357651493 0.0183372128982649 0.0151154602978625 0.0145225248902356 0.0140909485418917 0.0138327177533773 0.0138790538558903 0.0139332793888177 0.0140124160037074 0.0145233840715069 0.0157057873657242 0.0155340247452693 0.0134413587401672 0.0130828325119347 0.0128435724979935 0.0127389810938972 0.0126708818487862 0.0127456877906348 0.0128035979400575 0.0131690948255895 0.0137995389122503 0.0207996814653454 0.0207996814653454 0.0159698801733496 0.0159698801733496 0.0159698801733496 0.0159698801733496 0.0159698801733496 0.0159698801733496 0.0159698801733496 0.0159698801733496 0.0151875588315671 0.0145120772030942 0.0141358332322712 0.013922821969697 0.0139561078271969 0.0139260012753166 0.0140997661213288 0.0146115428038856 0.015835428135948 0.015835428135948 0.0135027295473501 0.0131055874729039 0.0129635571723677 0.0127418225363232 0.0127177145284622 0.0127144886363636 0.0128009420795534 0.013179496274602 0.0139089691213922 0.0139089691213922 0.0197077101487523 0.0183051399283096 0.017836144026278 0.0176340826717294 0.0175392137828468 0.017653585295909 0.017997224788924 0.0189836463418347 0.0212501110490647 0.0212501110490647 0.0150914254965963 0.0144570642924277 0.0141095850865661 0.0139102322410615 0.0139204473350254 0.0139519835065258 0.0140980950012182 0.0146462865031111 0.0159289340101523 0.0159289340101523 0.0134765545633711 0.0130817311109532 0.012866065855379 0.0126890655778486 0.0126837890248481 0.0127056039972195 0.0128159916378287 0.0132063704795588 0.0139864086732856 0.0139864086732856 0.0173312985677282 0.0173448656090845 0.0173647187960853 0.0174424050517235 0.0178919143610977 0.0191540488666829 0.0217179691309118 0.0217179691309118 0.0217179691309118 0.0217179691309118 0.014175165428682 0.013864302515478 0.0138441908353463 0.0138323153266255 0.0138818808911609 0.0141325249307606 0.0148236752166705 0.016411922564801 0.016411922564801 0.016411922564801 0.0132426180007739 0.0129211080029375 0.0126984713177917 0.0126731865099549 0.0126700754748595 0.0127234271097018 0.01287772057076 0.0133219707581326 0.0143314705595707 0.0143314705595707 0.0167975218155406 ...(+555 chars)])  InterpMethod=Cubic spline  InternalRulePriority=Speed  RndMeth=Simplest
      settings: InputPortMap=u0,u1,u2
  Simulink-PS Converter : nesl_utility/Simulink-PS Converter  PhysicalDomain=network_engine_domain  SubClassName=ps_input  LeftPortType=input  RightPortType=output  PseudoPeriodic=off  Frequencies=[]  NoiseDistribution=none  NoiseParameters=[]  Unit=1  AffineConversion=off  FilteringAndDerivatives=provide  SimscapeFilterOrder=1  InputFilterTimeConstant=0.001  UdotUserProvided=0
  SoC deployed calculator : Subsystem
  Variable Resistor : fl_lib/Electrical/Electrical Elements/Variable Resistor  Rmin=0 Ohm  thermalEnable=false  thermal_mass=1 J/K  i_specify=off  i_priority=None  i=0 A  i_nominal_specify=off  i_nominal_value=1  i_nominal_unit=A  v_specify=off  v_priority=None  v=0 V  v_nominal_specify=off  v_nominal_value=1  v_nominal_unit=V  T_specify=off  T_priority=None  T=300 K  T_nominal_specify=off  T_nominal_value=1  T_nominal_unit=K
  R_0 Output : PMIOPort  Side=Right
  R_0 Input : PMIOPort  Port=2  Side=Left
  wires:
  3-D Lookup Table/1 -> Simulink-PS Converter/1  "Resistance (ohms)"
  [pack_temp] -> 3-D Lookup Table/1  "Battery Temperature (C)"
  SoC deployed calculator/1(SoC Used (-)) -> 3-D Lookup Table/2  "SoC Used (-)"
  [pack_SOC] -> 3-D Lookup Table/3  "Battery C-Rate (1/h)"
  connections:
  Simulink-PS Converter/RConn1 -- Variable Resistor/LConn1
  Variable Resistor/LConn2 -- R_0 Input/RConn1
  Variable Resistor/RConn1 -- R_0 Output/RConn1

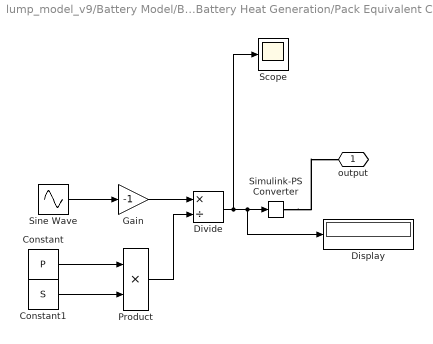
== system lump_model_v9/Battery Model/Battery Cells/Battery Heat Generation/Pack Equivalent Circuit Model/Sin Load ==
  Constant : Constant  Value=P
  Constant1 : Constant  Value=S
  Display : Display
  Divide : Product  Inputs=*/
  Gain : Gain  Gain=-1
  Product : Product
  Scope : Scope
  Simulink-PS Converter : nesl_utility/Simulink-PS Converter  PhysicalDomain=network_engine_domain  SubClassName=ps_input  LeftPortType=input  RightPortType=output  PseudoPeriodic=off  Frequencies=[]  NoiseDistribution=none  NoiseParameters=[]  Unit=J/s  AffineConversion=off  FilteringAndDerivatives=provide  SimscapeFilterOrder=1  InputFilterTimeConstant=0.001  UdotUserProvided=0
  Sine Wave : Sin  Amplitude=35000  Bias=-35000  SampleTime=0
  output : PMIOPort  Side=Right
  wires:
  Constant/1 -> Product/1
  Divide/1 -> Scope/1, Display/1, Simulink-PS Converter/1
  Product/1 -> Divide/2
  Constant1/1 -> Product/2
  Sine Wave/1 -> Gain/1
  Gain/1 -> Divide/1
  connections:
  Simulink-PS Converter/RConn1 -- output/RConn1

== system lump_model_v9/Battery Model/Battery Cells/Battery Heat Generation/Pack Equivalent Circuit Model/1 RC Branch Pair/Capacitor ==
  3-D Lookup Table : Lookup_n-D  NumberOfTableDimensions=3  BreakpointsForDimension1=[0 0.10000000000000001 0.20000000000000001 0.29999999999999999 0.40000000000000002 0.5 0.59999999999999998 0.69999999999999996 0.80000000000000004 0.90000000000000002]  BreakpointsForDimension2=[25 40 60]  BreakpointsForDimension3=[-9.61780450282953 -4.80898979382637 -0.960911970872145 -0.320367568578476 0.322065353393555 0.963286375388121 1.60506175114558 1.92546795576047]  Table=reshape([375048.648449974 1159.90322992473 951.997619966643 1023.52734053905 1264.66379771681 1218.91192846864 1324.16097822888 1324.16097822888 1324.16097822888 1324.16097822888 524831.6235963519 1405.79332031861 1069.22919322274 1175.14717943764 1367.23744100121 1260.55061265114 1207.99777638843 1364.09991275882 1364.09991275882 1364.09991275882 625952.677343929 1716.70628373224 1253.24601351832 1397.34444464425 1618.7833231449 1431.20308484048 1258.51579278261 1417.8301866691 1072.06296400368 1072.06296400368 571.436867621172 776.492599841087 753.2360807497161 751.662832923594 1000.58924291639 918.166575722267 880.777541964084 1246.20849208519 649.2656464158 649.2656464158 732.964321788551 917.222216669848 844.072444579772 854.007968237226 1173.64427163133 1054.09831129935 1011.54400364465 1278.60205976223 643.831380339981 401.679725383198 942.715839194136 1102.53007322919 1001.69989805492 1025.52091903243 1302.96604860053 1204.36098923799 1141.33303023627 1336.26018427124 632.000490105816 437.308871030655 497.519001559428 638.836101026978 620.196968289486 624.298651106496 926.612438694642 916.646626978831 919.540460315631 954.3479692922569 754.082032785149 482.696625229736 727.9477913594681 750.7211537141091 713.398561688199 726.41368533453 1098.92719349101 1038.93226856303 989.859609646585 1058.92879285714 794.014387499953 524.711993993523 970.156469311073 899.214507222865 833.612055893766 868.748380524749 1248.50515863718 1181.48655459494 1075.45646533421 1160.87304008035 853.313739847594 584.449762115293 602.591835881055 672.205592850799 645.053215858213 653.380582189803 944.177996833064 909.841400203883 929.765628919848 976.219717900361 754.7371862146319 494.217150084539 915.993597865675 775.710665648391 744.688179627271 764.279366391866 1083.94712392653 1052.9180026473 1056.17647774867 1048.26744202768 799.539039374876 531.354382027793 1179.81224264142 946.58112295029 871.625790849877 899.8612738476789 1252.67271787457 1190.18264415138 1143.15227156011 1146.99656340192 859.984161295439 591.100282805913 645.430130821415 645.430130821415 953.919996899601 953.919996899601 953.919996899601 953.919996899601 953.919996899601 953.919996899601 953.919996899601 953.919996899601 1042.50422156459 1042.50422156459 1042.50422156459 1042.50422156459 1042.50422156459 1042.50422156459 1042.50422156459 502.078889842115 502.078889842115 502.078889842115 862.408886305344 862.408886305344 879.993881307122 879.993881307122 879.993881307122 1151.75841568185 1114.77161556301 837.449976374495 837.449976374495 837.449976374495 704.730084085008 682.883476175586 633.395058953854 927.032274622301 903.57556617401 937.530313755239 1004.66873517708 699.096851693738 438.536846421278 953.919996899601 796.71670204175 757.678503338422 711.674997132905 1018.11208179599 968.358710460414 1067.83602239428 1079.67154814756 733.271792259711 473.273991427527 473.273991427527 946.983348910683 887.161835934911 849.286896538658 1146.15975240705 1054.30384186608 1214.81250987349 1121.31894344376 801.259977023257 520.593227330271 520.593227330271 1036.48768981613 935.984338919748 905.638209501089 976.810559897871 997.134452545195 641.452357535268 411.212851248204 411.212851248204 411.212851248204 411.212851248204 835.686630005248 1333.88129096757 1075.54617197992 1040.21406918774 1069.45351947977 1053.40584629504 683.422653905484 417.697711241573 417.697711241573 417.697711241573 1081.14414911427 1011.25789762967 1736.55389506661 1133.750291248 1213.03383422998 1176.13981811032 1118.89742557524 734.7075758805061 452.760818938771 452.760818938771 991.292097729902 928.455308273977 945.857314973298 1104.0340737638 902.22563646243 574.750569618313 377.638239434614 377.638239434614 377.638239434614 377.638239434614 1110.38063825923 1059.53727862117 1010.25884842023 1291.74503680783 892.84888765341 590.78684552854 377.294781616954 377.294781616954 377.294781616954 377.294781616954 1069.26947841736 1321.11271537775 1150.36267367768 1113.47214095653 1651.66945871112 773.347976877209 611.426949020729 372.349693751735 372.349693751735 372.349693751735], [10 3 8])  InterpMethod=Cubic spline  InternalRulePriority=Speed  RndMeth=Simplest
      settings: InputPortMap=u0,u1,u2
  Gain : Gain  Gain=C_nominal
  Simulink-PS Converter : nesl_utility/Simulink-PS Converter  PhysicalDomain=network_engine_domain  SubClassName=ps_input  LeftPortType=input  RightPortType=output  PseudoPeriodic=off  Frequencies=[]  NoiseDistribution=none  NoiseParameters=[]  Unit=1  AffineConversion=off  FilteringAndDerivatives=provide  SimscapeFilterOrder=1  InputFilterTimeConstant=0.001  UdotUserProvided=0
  SoC deployed calculator : Subsystem
  Variable Capacitor : ee_lib/Passive/Variable Capacitor  prm=2  Cmin=1e-9 F  r=1e-6 Ohm  v0=0 V  q0=0 C
      settings: InternalSimscapePortConfiguration="{\"Bottom\":[],\"Left\":[{\"id\":\"C\",\"label\":\"C\",\"type\":\"input\"},{\"id\":\"p\",\"label\":\"+\",\"type\":\"foundation.electrical.electrical\"}],\"Right\":[{\"id\":\"n\",\"label\":\"-\",\"type\":\"foundation.electrical.electrical\"}],\"Top\":[]}"
  Capacitor Output : PMIOPort  Side=Right
  Capacitor Input : PMIOPort  Port=2  Side=Left
  wires:
  [pack_temp] -> 3-D Lookup Table/1  "Battery Temperature (C)"
  3-D Lookup Table/1 -> Simulink-PS Converter/1  "Capacitance (F)"
  SoC deployed calculator/1(SoC Used (-)) -> 3-D Lookup Table/2  "SoC Used (-)"
  Gain/1 -> 3-D Lookup Table/3  "Battery C-Rate (1/h)"
  [pack_current] -> Gain/1  "Battery Current (A)"
  connections:
  Variable Capacitor/LConn1 -- Simulink-PS Converter/RConn1
  Variable Capacitor/LConn2 -- Capacitor Input/RConn1
  Variable Capacitor/RConn1 -- Capacitor Output/RConn1

== system lump_model_v9/Battery Model/Battery Cells/Battery Heat Generation/Pack Equivalent Circuit Model/1 RC Branch Pair/Resistor ==
  3-D Lookup Table : Lookup_n-D  NumberOfTableDimensions=3  BreakpointsForDimension1=[0 0.10000000000000001 0.20000000000000001 0.29999999999999999 0.40000000000000002 0.5 0.59999999999999998 0.69999999999999996 0.80000000000000004 0.90000000000000002]  BreakpointsForDimension2=[25 40 60]  BreakpointsForDimension3=[-9.61780450282953 -4.80898979382637 -0.960911970872145 -0.320367568578476 0.322065353393555 0.963286375388121 1.60506175114558 1.92546795576047]  Table=reshape([0.00588147412977802 0.00771600435781647 0.009828390456229611 0.0101584233330109 0.0119638079081804 0.0127715726618859 0.017971482863859 0.017971482863859 0.017971482863859 0.017971482863859 0.00675271639946551 0.00844670653735221 0.00988815160847021 0.00994305533616506 0.0115110358012954 0.011707491117447 0.0130991082277302 0.0204976331005528 0.0204976331005528 0.0204976331005528 0.00659227972306084 0.00777517089719098 0.00916168262401082 0.0090932583049207 0.0109662634135486 0.0107852654316738 0.010862069104398 0.0136715597119813 0.0260710399310775 0.0260710399310775 0.0102639573164867 0.00958566696060849 0.0134274828406036 0.0121919644393604 0.012574983051026 0.0139650502124618 0.0134138732057371 0.0217425517438959 0.0434178054727066 0.0434178054727066 0.009868636372700371 0.00848567662538143 0.0119963346205773 0.0107974658447741 0.0116195010710329 0.0130222466600467 0.012077754176894 0.0171190523265226 0.0244118313220914 0.037863629881143 0.00912676416017431 0.00696286240573036 0.0102977048011881 0.009196352746627119 0.0102141213545697 0.0119626314179404 0.0107778047334625 0.013680896040741 0.0175873956759502 0.0245980383098257 0.0215184848783088 0.0183923910278187 0.0250351781309079 0.0242940594144215 0.0158147625807696 0.0191247772781543 0.0195295463260478 0.0153707177627115 0.0511295288689729 0.11963129851428 0.0170740987724351 0.0136990667619507 0.0203323921306775 0.020911864667035 0.0131024141512807 0.0163327432065457 0.0154905336807582 0.0126982783221291 0.0417927372497635 0.09448030318342771 0.0144305907620296 0.00963593452127621 0.0159213175984991 0.0175291982490748 0.0110124395314545 0.014303919148238 0.0123312290724997 0.0107725367483906 0.0369779367056412 0.0846365661929343 0.0248851733831933 0.0207841511557094 0.0300378353175187 0.033391493573513 0.0170836078110103 0.0201199135069218 0.0206371148284127 0.019353693086831 0.0463135641879321 0.094847712688643 0.0197702140742291 0.0144116185181984 0.0222044657120929 0.0259842766925567 0.0137843989199457 0.0166623651363753 0.0175876801522339 0.0168136535538863 0.038284582163463 0.0908603837464433 0.0167411776922126 0.009996673804255811 0.0162657013962451 0.020174222042422 0.0116149612925061 0.0143195261592052 0.0150672271897213 0.0148098870664063 0.0341633722357047 0.0862713177190066 0.0207996814653454 0.0207996814653454 0.0159698801733496 0.0159698801733496 0.0159698801733496 0.0159698801733496 0.0159698801733496 0.0159698801733496 0.0159698801733496 0.0159698801733496 0.0133651748626512 0.0133651748626512 0.0133651748626512 0.0133651748626512 0.0133651748626512 0.0133651748626512 0.0133651748626512 0.07476659702696239 0.07476659702696239 0.07476659702696239 0.0132948216388165 0.0132948216388165 0.0149410842576491 0.0149410842576491 0.0149410842576491 0.0150770393806212 0.011909387273048 0.0322321993634374 0.0322321993634374 0.0322321993634374 0.0132057977190401 0.0156490707143108 0.0178262558410046 0.0139516187042768 0.0167853371590393 0.0194991262247213 0.0138756790305067 0.0377636919354958 0.0612629201714896 0.0612629201714896 0.00938277845805918 0.0122314968566107 0.0135938888162443 0.0106085347083951 0.0134728950804437 0.0174238605970247 0.0109849250430613 0.0334727272756119 0.0569930094590715 0.0569930094590715 0.00693155638131778 0.009719336616209041 0.0109385133708481 0.00847750902210259 0.0107105188807283 0.0151914213162909 0.009203850214382241 0.0304373318921658 0.0530686867032268 0.0530686867032268 0.0145311241759147 0.0133786081559239 0.0159661102708986 0.0178626567723149 0.0123286521657843 0.0335537337822512 0.0507022576571237 0.0507022576571237 0.0507022576571237 0.0507022576571237 0.0123185256294987 0.0131796038887959 0.01094939395699 0.0127699708123327 0.0156064836229331 0.0100916669836755 0.0303633624297924 0.0471555442124812 0.0471555442124812 0.0471555442124812 0.00608477059693291 0.00971622930003458 0.0117436517796757 0.00848843783550436 0.0115592708056212 0.0137664319684855 0.008616880649104999 0.0281554798738857 0.0431640134009286 ...(+601 chars)])  InterpMethod=Cubic spline  InternalRulePriority=Speed  RndMeth=Simplest
      settings: InputPortMap=u0,u1,u2
  Gain : Gain  Gain=C_nominal
  Simulink-PS Converter : nesl_utility/Simulink-PS Converter  PhysicalDomain=network_engine_domain  SubClassName=ps_input  LeftPortType=input  RightPortType=output  PseudoPeriodic=off  Frequencies=[]  NoiseDistribution=none  NoiseParameters=[]  Unit=1  AffineConversion=off  FilteringAndDerivatives=provide  SimscapeFilterOrder=1  InputFilterTimeConstant=0.001  UdotUserProvided=0
  SoC deployed calculator : Subsystem
  Variable Resistor : fl_lib/Electrical/Electrical Elements/Variable Resistor  Rmin=0 Ohm  thermalEnable=false  thermal_mass=1 J/K  i_specify=off  i_priority=None  i=0 A  i_nominal_specify=off  i_nominal_value=1  i_nominal_unit=A  v_specify=off  v_priority=None  v=0 V  v_nominal_specify=off  v_nominal_value=1  v_nominal_unit=V  T_specify=off  T_priority=None  T=300 K  T_nominal_specify=off  T_nominal_value=1  T_nominal_unit=K
  Resistor Output : PMIOPort  Side=Right
  Resistor Input : PMIOPort  Port=2  Side=Left
  wires:
  3-D Lookup Table/1 -> Simulink-PS Converter/1  "Resistance (ohms)"
  [pack_temp] -> 3-D Lookup Table/1  "Battery Temperature (C)"
  SoC deployed calculator/1(SoC Used (-)) -> 3-D Lookup Table/2  "SoC Used (-)"
  [pack_current] -> Gain/1  "Battery Current (A)"
  Gain/1 -> 3-D Lookup Table/3  "Battery C-Rate (1/h)"
  connections:
  Simulink-PS Converter/RConn1 -- Variable Resistor/LConn1
  Variable Resistor/LConn2 -- Resistor Input/RConn1
  Variable Resistor/RConn1 -- Resistor Output/RConn1

== system lump_model_v9/Battery Model/Battery Cells/Battery Heat Generation/Pack Equivalent Circuit Model/OCV/SoC deployed calculator ==
  Constant : Constant  Value=SoC_initial
  Sum : Sum  Inputs=|+-
  SoC Used (-) : Outport
  wires:
  [pack_SOC] -> Sum/2  "Battery SoC (-)"
  Sum/1 -> SoC Used (-)/1
  Constant/1 -> Sum/1

== system lump_model_v9/Battery Model/Battery Cells/Battery Heat Generation/Pack Equivalent Circuit Model/R_0 Resistor/SoC deployed calculator ==
  Constant : Constant  Value=SoC_initial
  Sum : Sum  Inputs=|+-
  SoC Used (-) : Outport
  wires:
  [pack_SOC] -> Sum/2  "Battery SoC (-)"
  Sum/1 -> SoC Used (-)/1
  Constant/1 -> Sum/1

== system lump_model_v9/Battery Model/Battery Cells/Battery Heat Generation/Pack Equivalent Circuit Model/1 RC Branch Pair/Capacitor/SoC deployed calculator ==
  Constant : Constant  Value=SoC_initial
  Sum : Sum  Inputs=|+-
  SoC Used (-) : Outport
  wires:
  [pack_SOC] -> Sum/2  "Battery SoC (-)"
  Sum/1 -> SoC Used (-)/1
  Constant/1 -> Sum/1

== system lump_model_v9/Battery Model/Battery Cells/Battery Heat Generation/Pack Equivalent Circuit Model/1 RC Branch Pair/Resistor/SoC deployed calculator ==
  Constant : Constant  Value=SoC_initial
  Sum : Sum  Inputs=|+-
  SoC Used (-) : Outport
  wires:
  [pack_SOC] -> Sum/2  "Battery SoC (-)"
  Sum/1 -> SoC Used (-)/1
  Constant/1 -> Sum/1
